simulink model "CTRNNSLSF"  (R2017a)
settings: Solver=VariableStepAuto  StartTime=0.0  StopTime=50.0  RelTol=1e-3
libraries: simulink x5
settings Model: Creator=musaup  LastModifiedBy=musaup

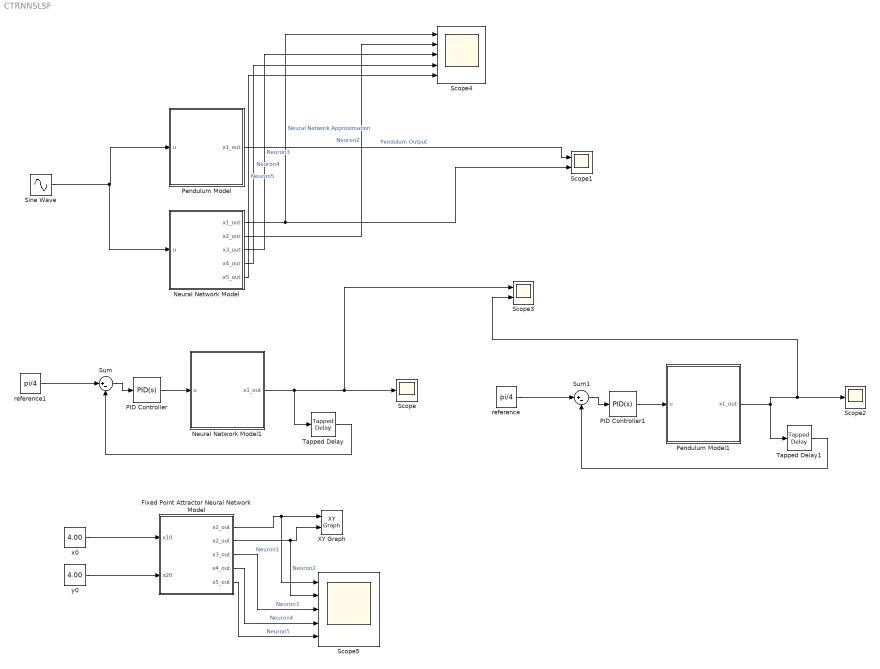
== system CTRNNSLSF ==
  Fixed Point Attractor Neural Network Model : Stateflow chart  TreatAsAtomicUnit=on
  Neural Network Model : Stateflow chart  TreatAsAtomicUnit=on
  Neural Network Model1 : Stateflow chart  TreatAsAtomicUnit=on
  PID Controller : simulink/Continuous/PID Controller  Controller=PID  TimeDomain=Continuous-time  SampleTime=-1  IntegratorMethod=Forward Euler  FilterMethod=Forward Euler  Form=Parallel  UseFilter=on  ControllerParametersSource=internal  P=149.944875551697  I=175.606429824802  D=28.3552517737635  N=97.9428951201381  InitialConditionSource=internal  InitialConditionForIntegrator=0  InitialConditionForFilter=0  ExternalReset=none  LimitOutput=off  UpperSaturationLimit=inf  LowerSaturationLimit=-inf  LinearizeAsGain=on  AntiWindupMode=none  Kb=1  TrackingMode=off  Kt=1  PParamMin=[]  PParamMax=[]  IParamMin=[]  IParamMax=[]  DParamMin=[]  DParamMax=[]  NParamMin=[]  NParamMax=[]  KbParamMin=[]  KbParamMax=[]  KtParamMin=[]  KtParamMax=[]  POutMin=[]  POutMax=[]  IOutMin=[]  IOutMax=[]  DOutMin=[]  DOutMax=[]  NOutMin=[]  NOutMax=[]  KbOutMin=[]  KbOutMax=[]  KtOutMin=[]  KtOutMax=[]  IntegratorOutMin=[]  IntegratorOutMax=[]  FilterOutMin=[]  FilterOutMax=[]  SumOutMin=[]  SumOutMax=[]  SumI1OutMin=[]  SumI1OutMax=[]  SumI2OutMin=[]  SumI2OutMax=[]  SumI3OutMin=[]  SumI3OutMax=[]  SumDOutMin=[]  SumDOutMax=[]  SaturationOutMin=[]  SaturationOutMax=[]  IntegratorContinuousStateAttributes=''  IntegratorStateMustResolveToSignalObject=off  IntegratorRTWStateStorageClass=Auto  FilterContinuousStateAttributes=''  FilterStateMustResolveToSignalObject=off  FilterRTWStateStorageClass=Auto  DifferentiatorICPrevScaledInput=0  DifferentiatorOutMin=[]  DifferentiatorOutMax=[]  InitialConditionSetting=State (most efficient)
  PID Controller1 : simulink/Continuous/PID Controller  Controller=PID  TimeDomain=Continuous-time  SampleTime=-1  IntegratorMethod=Forward Euler  FilterMethod=Forward Euler  Form=Parallel  UseFilter=on  ControllerParametersSource=internal  P=149.944875420298  I=175.606429689668  D=28.3552517551584  N=97.9428950591106  InitialConditionSource=internal  InitialConditionForIntegrator=0  InitialConditionForFilter=0  ExternalReset=none  LimitOutput=off  UpperSaturationLimit=inf  LowerSaturationLimit=-inf  LinearizeAsGain=on  AntiWindupMode=none  Kb=1  TrackingMode=off  Kt=1  PParamMin=[]  PParamMax=[]  IParamMin=[]  IParamMax=[]  DParamMin=[]  DParamMax=[]  NParamMin=[]  NParamMax=[]  KbParamMin=[]  KbParamMax=[]  KtParamMin=[]  KtParamMax=[]  POutMin=[]  POutMax=[]  IOutMin=[]  IOutMax=[]  DOutMin=[]  DOutMax=[]  NOutMin=[]  NOutMax=[]  KbOutMin=[]  KbOutMax=[]  KtOutMin=[]  KtOutMax=[]  IntegratorOutMin=[]  IntegratorOutMax=[]  FilterOutMin=[]  FilterOutMax=[]  SumOutMin=[]  SumOutMax=[]  SumI1OutMin=[]  SumI1OutMax=[]  SumI2OutMin=[]  SumI2OutMax=[]  SumI3OutMin=[]  SumI3OutMax=[]  SumDOutMin=[]  SumDOutMax=[]  SaturationOutMin=[]  SaturationOutMax=[]  IntegratorContinuousStateAttributes=''  IntegratorStateMustResolveToSignalObject=off  IntegratorRTWStateStorageClass=Auto  FilterContinuousStateAttributes=''  FilterStateMustResolveToSignalObject=off  FilterRTWStateStorageClass=Auto  DifferentiatorICPrevScaledInput=0  DifferentiatorOutMin=[]  DifferentiatorOutMax=[]  InitialConditionSetting=State (most efficient)
  Pendulum Model : Stateflow chart  TreatAsAtomicUnit=on
  Pendulum Model1 : Stateflow chart  TreatAsAtomicUnit=on
  Scope : Scope
  Scope1 : Scope  NumInputPorts=2
  Scope2 : Scope
  Scope3 : Scope  NumInputPorts=2
  Scope4 : Scope  NumInputPorts=5
  Scope5 : Scope  NumInputPorts=5
  Sine Wave : Sin  Amplitude=pi/2  Frequency=(2*pi)/12.5  SampleTime=0
  Sum : Sum  Inputs=|+-
  Sum1 : Sum  Inputs=|+-
  Tapped Delay : simulink/Discrete/Tapped Delay  vinit=0  samptime=0.01  NumDelays=1  DelayOrder=Oldest  includeCurrent=off
  Tapped Delay1 : simulink/Discrete/Tapped Delay  vinit=0  samptime=0.01  NumDelays=1  DelayOrder=Oldest  includeCurrent=off
  XY Graph : simulink/Sinks/XY Graph  xmin=-1  xmax=1  ymin=-1  ymax=1  st=-1
  reference : Constant  Value=pi/4
  reference1 : Constant  Value=pi/4
  x0 : Constant  Value=4.00
  y0 : Constant  Value=4.00
  wires:
  Pendulum Model/1(x1_out) -> Scope1/1  "Pendulum Output"
  Neural Network Model/1(x1_out) -> Scope4/1, Scope1/2  "Neural Network Approximation"
  Sine Wave/1 -> Neural Network Model/1(u), Pendulum Model/1(u)
  Neural Network Model1/1(x1_out) -> Tapped Delay/1, Scope3/1, Scope/1
  reference1/1 -> Sum/1
  Sum/1 -> PID Controller/1
  PID Controller/1 -> Neural Network Model1/1(u)
  Tapped Delay/1 -> Sum/2
  PID Controller1/1 -> Pendulum Model1/1(u)
  Tapped Delay1/1 -> Sum1/2
  reference/1 -> Sum1/1
  Sum1/1 -> PID Controller1/1
  Pendulum Model1/1(x1_out) -> Tapped Delay1/1, Scope3/2, Scope2/1
  Neural Network Model/2(x2_out) -> Scope4/2  "Neuron2"
  Neural Network Model/3(x3_out) -> Scope4/3  "Neuron3"
  Neural Network Model/4(x4_out) -> Scope4/4  "Neuron4"
  Neural Network Model/5(x5_out) -> Scope4/5  "Neuron5"
  Fixed Point Attractor Neural Network Model/1(x1_out) -> Scope5/1, XY Graph/1  "Neuron1"
  Fixed Point Attractor Neural Network Model/2(x2_out) -> Scope5/2, XY Graph/2  "Neuron2"
  Fixed Point Attractor Neural Network Model/3(x3_out) -> Scope5/3  "Neuron3"
  Fixed Point Attractor Neural Network Model/4(x4_out) -> Scope5/4  "Neuron4"
  Fixed Point Attractor Neural Network Model/5(x5_out) -> Scope5/5  "Neuron5"
  x0/1 -> Fixed Point Attractor Neural Network Model/1(x10)
  y0/1 -> Fixed Point Attractor Neural Network Model/2(x20)

== stateflow chart CTRNNSLSF/Pendulum Model ==
  settings: updateMethod=CONTINUOUS  executeAtInitialization=1  initializeOutput=1
  state Pendulum
    du:
    % derivatives
    x1_dot = x2;
    x2_dot = -9.81*x1-0.5*x2+0.5*u;
    % outputs
    x1_out = x1;
  (default) -> Pendulum : {
      | x1 = 0;
      | x2 = 0;
      | }
  data: u input; x1 local; x2 local; x1_out output
  data x1 settings: updateMethod=SF_CONTINUOUS_TIME_DATA
  data x2 settings: updateMethod=SF_CONTINUOUS_TIME_DATA

== stateflow chart CTRNNSLSF/Neural Network Model ==
  settings: updateMethod=CONTINUOUS  executeAtInitialization=1  initializeOutput=1
  state DFPRNN
    du:
    % derivatives
    x1_dot=-x1+0.4684*tanh(x1)-2.4995*tanh(x2) +0.4211*tanh(x3) -0.2848*tanh(x4) +0.1995*tanh(x5)+0.0050*u;
    x2_dot=-x2+1.3615*tanh(x1)+0.0642*tanh(x2) + 0.0413*tanh(x3) - 1.8925*tanh(x4) - 1.6608*tanh(x5)-0.2111*u;
    x3_dot=-x3-0.8185*tanh(x1)-0.9241*tanh(x2)-0.0743*tanh(x3) -0.1264*tanh(x4) +0.1484*tanh(x5)+0.1689*u;
    x4_dot=-x4-0.3257*tanh(x1)+1.2319*tanh(x2)-1.0997*tanh(x3) +0.2192*tanh(x4) -0.8547*tanh(x5)+0.0645*u;
    x5_dot=-x5-1.2444*tanh(x1) + 0.4396*tanh(x2) - 0.5466*tanh(x3) + 1.7342*tanh(x4) - 0.5953*tanh(x5)-0.0413*u;
    % outputs
    x1_out = x1;
    x2_out=x2;
    x3_out=x3;
    x4_out=x4;
    x5_out=x5;
  (default) -> DFPRNN : {x1 = -0.0097;
      | x2= -0.0065;
      | x3=0.0171;
      | x4=-0.0097;
      | x5= 0.0025;
      | }
  data: u input; x1 local; x2 local; x3 local; x4 local; x5 local; x1_out output; x2_out output; x3_out output; x4_out output; x5_out output
  data x1 settings: updateMethod=SF_CONTINUOUS_TIME_DATA
  data x2 settings: updateMethod=SF_CONTINUOUS_TIME_DATA
  data x3 settings: updateMethod=SF_CONTINUOUS_TIME_DATA
  data x4 settings: updateMethod=SF_CONTINUOUS_TIME_DATA
  data x5 settings: updateMethod=SF_CONTINUOUS_TIME_DATA

== stateflow chart CTRNNSLSF/Neural Network Model1 ==
  settings: updateMethod=CONTINUOUS  executeAtInitialization=1  initializeOutput=1
  state Falling
    du:
    % derivatives
    x1_dot=-x1+0.4684*tanh(x1)-2.4995*tanh(x2) +0.4211*tanh(x3) -0.2848*tanh(x4) +0.1995*tanh(x5)+0.0050*u;
    x2_dot=-x2+1.3615*tanh(x1)+0.0642*tanh(x2) + 0.0413*tanh(x3) - 1.8925*tanh(x4) - 1.6608*tanh(x5)-0.2111*u;
    x3_dot=-x3-0.8185*tanh(x1)-0.9241*tanh(x2)-0.0743*tanh(x3) -0.1264*tanh(x4) +0.1484*tanh(x5)+0.1689*u;
    x4_dot=-x4-0.3257*tanh(x1)+1.2319*tanh(x2)-1.0997*tanh(x3) +0.2192*tanh(x4) -0.8547*tanh(x5)+0.0645*u;
    x5_dot=-x5-1.2444*tanh(x1) + 0.4396*tanh(x2) - 0.5466*tanh(x3) + 1.7342*tanh(x4) - 0.5953*tanh(x5)-0.0413*u;
    % outputs
    x1_out = x1;
  (default) -> Falling : {
      | x1 = -0.0097;
      | x2= -0.0065;
      | x3=0.0171;
      | x4=-0.0097;
      | x5= 0.0025;
      |
      | }
  data: u input; x1 local; x2 local; x3 local; x4 local; x5 local; x1_out output
  data x1 settings: updateMethod=SF_CONTINUOUS_TIME_DATA
  data x2 settings: updateMethod=SF_CONTINUOUS_TIME_DATA
  data x3 settings: updateMethod=SF_CONTINUOUS_TIME_DATA
  data x4 settings: updateMethod=SF_CONTINUOUS_TIME_DATA
  data x5 settings: updateMethod=SF_CONTINUOUS_TIME_DATA

== stateflow chart CTRNNSLSF/Pendulum Model1 ==
  settings: updateMethod=CONTINUOUS  executeAtInitialization=1  initializeOutput=1
  state Falling
    du:
    % derivatives
    x1_dot = x2;
    x2_dot = -9.81*x1-0.5*x2+0.5*u;
    % outputs
    x1_out = x1;
  (default) -> Falling : {
      | x1 = 0;
      | x2 = 0;
      | }
  data: u input; x1 local; x2 local; x1_out output
  data x1 settings: updateMethod=SF_CONTINUOUS_TIME_DATA
  data x2 settings: updateMethod=SF_CONTINUOUS_TIME_DATA

== stateflow chart CTRNNSLSF/Fixed Point Attractor Neural Network Model ==
  settings: updateMethod=CONTINUOUS  executeAtInitialization=1  initializeOutput=1
  state Falling
    du:
    % derivatives
    x1_dot=-(10^-6)*x1 -1.2033*tanh(x3) -0.0720*tanh(x4) -0.9364*tanh(x5);
    x2_dot=-(10^-6)*x2+ 1.1881*tanh(x3) - 1.5002*tanh(x4) +0.9352*tanh(x5);
    x3_dot=-(10^-6)*x3-1.5863*tanh(x3) +0.0701*tanh(x4) -1.2355*tanh(x5);
    x4_dot=-(10^-6)*x4+0.0857*tanh(x3) -0.2995*tanh(x4) +0.0687*tanh(x5);
    x5_dot=-(10^-6)*x5+1.7898*tanh(x3) - 0.0846*tanh(x4) + 1.3940*tanh(x5);
    % outputs
    x1_out = x1;
    x2_out = x2;
    x3_out = x3;
    x4_out = x4;
    x5_out = x5;
  (default) -> Falling : {
      | x1 =x10;
      | x2=x20;
      | x3=1.2146*x10 - 0.105*x20-(7.564900000000000*(10^-5));
      | x4=0.1202*x10 + 0.1939*x20+(1.347080000000000*(10^(-4)));
      | x5=-1.367*x10 + 0.122*x20-(6.249250000000000*(10^(-6)))
      |
      | }
  data: x1 local; x2 local; x3 local; x4 local; x5 local; x1_out output; x2_out output; x3_out output; x4_out output; x5_out output; x10 input; x20 input
  data x1 settings: updateMethod=SF_CONTINUOUS_TIME_DATA
  data x2 settings: updateMethod=SF_CONTINUOUS_TIME_DATA
  data x3 settings: updateMethod=SF_CONTINUOUS_TIME_DATA
  data x4 settings: updateMethod=SF_CONTINUOUS_TIME_DATA
  data x5 settings: updateMethod=SF_CONTINUOUS_TIME_DATA
